simulink model "asm1_w_primclar"  (R2023b)
settings: Solver=ode15s  StartTime=0.0  StopTime=200  FixedStep=0.01  RelTol=1e-5  AbsTol=1e-8
undefined symbols (not defined in the file): PAR1, PAR_P, T, TEMPMODEL, VOL_P, XINIT_P, XINITDELAYPRIMARY, XVEKTOR_P
settings Model: Creator=ielulf  LastModifiedBy=BuB
settings SolverCC: AutoScaleAbsTol=off  AlgebraicLoopSolver=TrustRegion
settings DataIOCC: InitialState=xFinal  SaveFormat=Array  SignalLoggingSaveFormat=ModelDataLogs  SaveOutput=off  ReturnWorkspaceOutputs=off  TimeSaveName=t  SignalLoggingName=sigsOut  OutputTimes=[0:(1/96):609]
settings OptimizationCC: BlockReduction=off  BooleanDataType=off  OptimizeBlockIOStorage=off  BufferReuse=off  GlobalBufferReuse=off  ExpressionFolding=off  LocalBlockOutputs=off  InitFltsAndDblsToZero=on  LifeSpan=inf  OptimizeDataStoreBuffers=off  BusAssignmentInplaceUpdate=off
settings DebuggingCC: SaveWithParameterizedLinksMsg=none  UnderspecifiedInitializationDetection=Classic  MergeDetectMultiDrivingBlocksExec=none  SignalResolutionControl=TryResolveAllWithWarning  InheritedTsInSrcMsg=none  MultiTaskDSMMsg=warning  MultiTaskCondExecSysMsg=none  FcnCallInpInsideContextMsg=warning  UnconnectedInputMsg=warning  UnconnectedLineMsg=warning  SFUnexpectedBacktrackingDiag=warning  SFNoUnconditionalDefaultTransitionDiag=warning  SFExecutionAtInitializationDiag=none  ArithmeticOperatorsInVariantConditions=warning
settings HardwareCC: ProdBitPerPointer=32  ProdBitPerSizeT=32  ProdBitPerPtrDiffT=32  ProdLargestAtomicFloat=None  ProdIntDivRoundTo=Undefined  ProdEndianess=Unspecified  ProdWordSize=32  ProdHWDeviceType=32-bit Generic  TargetUnknown=on
settings ModelReferenceCC: EnableRefExpFcnMdlSchedulingChecks=on  PropagateSignalLabelsOutOfModel=off
settings RTWCC: TemplateMakefile=grt_unix.tmf
settings CodeAppCC: StateflowObjectComments=on
settings GRTTargetCC: TargetFcnLib=ansi_tfl_tmw.mat  TargetLangStandard=C89/C90 (ANSI)  CombineOutputUpdateFcns=off  GRTInterface=on
settings ConfigComp: CovMetricSettings=dw  CovSaveCumulativeToWorkspaceVar=on  CovSaveSingleToWorkspaceVar=on

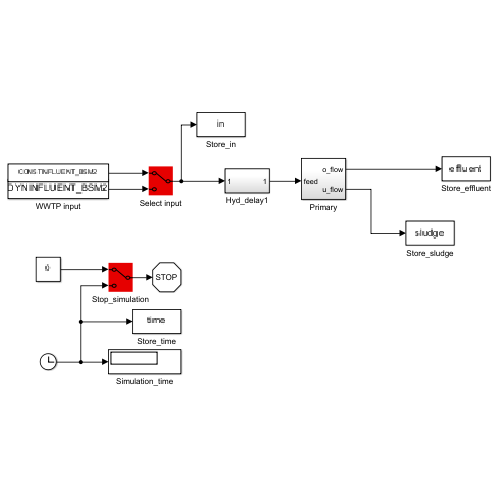
[thumbnail: Simulink's stored preview of the top-level diagram]
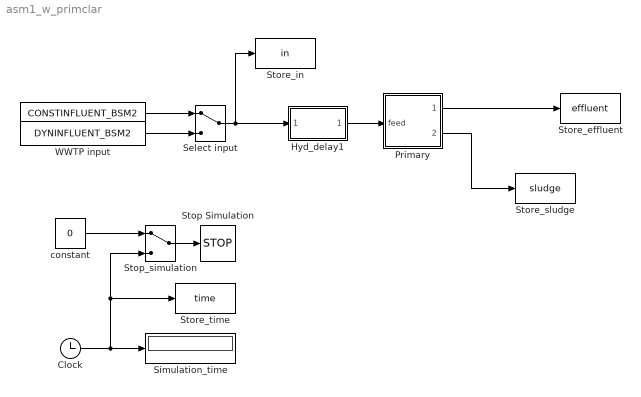
== system asm1_w_primclar ==
  " " : FromWorkspace  VariableName=CONSTINFLUENT_BSM2  SampleTime=-1  ZeroCross=off  OutputAfterFinalValue=Holding final value
  " constant" : Constant  Value=0
  Clock : Clock
  Hyd_delay1 : Subsystem
  Primary : Subsystem
  Select input : ManualSwitch
  Simulation_time : Display
  Stop Simulation : Stop
  Stop_simulation : ManualSwitch
  Store_effluent : ToWorkspace  VariableName=effluent
  Store_in : ToWorkspace  VariableName=in
  Store_sludge : ToWorkspace  VariableName=sludge
  Store_time : ToWorkspace  VariableName=time
  WWTP input : FromWorkspace  VariableName=DYNINFLUENT_BSM2  SampleTime=-1  ZeroCross=off  OutputAfterFinalValue=Holding final value
  wires:
  Primary/1(o_flow) -> Store_effluent/1
  Clock/1 -> Simulation_time/1, Stop_simulation/2, Store_time/1
  Stop_simulation/1 -> Stop Simulation/1
  " constant"/1 -> Stop_simulation/1
  " "/1 -> Select input/1
  WWTP input/1 -> Select input/2
  Select input/1 -> Hyd_delay1/1(Input), Store_in/1
  Hyd_delay1/1(Output) -> Primary/1(feed)
  Primary/2(u_flow) -> Store_sludge/1

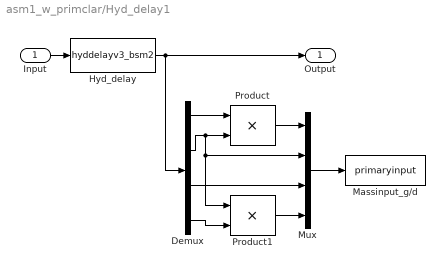
== system asm1_w_primclar/Hyd_delay1 ==
  Input : Inport
  Demux : Demux  Outputs=[14,1,1,5]
      settings: DisplayOption=none
  Hyd_delay : S-Function  FunctionName=hyddelayv3_bsm2  Parameters=XINITDELAYPRIMARY,PAR1,T  SFunctionDeploymentMode=off  EnableBusSupport=off
  Massinput_g/d : ToWorkspace  VariableName=primaryinput  SampleTime=-1
  Mux : Mux
  Product : Product  SaturateOnIntegerOverflow=on  OutDataTypeStr=Inherit: Same as first input
  Product1 : Product  SaturateOnIntegerOverflow=on  OutDataTypeStr=Inherit: Same as first input
  Output : Outport
  wires:
  Demux/4 -> Product1/2
  Product1/1 -> Mux/4
  Demux/3 -> Mux/3
  Demux/2 -> Product1/1, Mux/2, Product/2
  Input/1 -> Hyd_delay/1
  Hyd_delay/1 -> Demux/1, Output/1
  Demux/1 -> Product/1
  Product/1 -> Mux/1
  Mux/1 -> Massinput_g/d/1

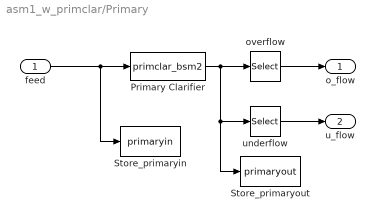
== system asm1_w_primclar/Primary ==
  feed : Inport
  Primary Clarifier : S-Function  FunctionName=primclar_bsm2  Parameters=XINIT_P,XVEKTOR_P,PAR_P,VOL_P,PAR1,TEMPMODEL  SFunctionDeploymentMode=off  EnableBusSupport=off
  Store_primaryin : ToWorkspace  VariableName=primaryin
  Store_primaryout : ToWorkspace  VariableName=primaryout
  overflow : Selector  InputPortWidth=63  IndexOptions=Index vector (dialog)  Indices=[1:21]  OutputSizes=1
  underflow : Selector  InputPortWidth=63  IndexOptions=Index vector (dialog)  Indices=[22:42]  OutputSizes=1
  o_flow : Outport
  u_flow : Outport  Port=2
  wires:
  Primary Clarifier/1 -> Store_primaryout/1, underflow/1, overflow/1
  feed/1 -> Primary Clarifier/1, Store_primaryin/1
  underflow/1 -> u_flow/1
  overflow/1 -> o_flow/1
